simulink model "HANcoder_E407_DYS_MP"  (R2018b)
settings: Solver=FixedStepDiscrete  StartTime=0.0  StopTime=1  FixedStep=0.01  RelTol=1e-3
PreLoadFcn:
  | librarySetup
  | eval([bdroot,'_startup']) %Calling [modelName]_startup.m
values from neighbouring files (symbols this model uses):
  basic_cycle_duration_bc0 = TM_Reset_Board   + COMP_duration    (= 212)    [HANcoder_E407_DYS_MP_startup.m]
  basic_cycle_duration_bc1 = basic_cycle_duration_bc0    (= 212)    [HANcoder_E407_DYS_MP_startup.m]
  comm_delay_estimation1 = round(comm_delay_measured1*hardware_granularity/frequency_IRQ)    [HANcoder_E407_DYS_MP_startup.m]
  comm_delay_estimation2 = round(comm_delay_measured2*hardware_granularity/frequency_IRQ)    [HANcoder_E407_DYS_MP_startup.m]
  COMM_Phase1 = Simulink.Parameter    [HANcoder_E407_DYS_MP_startup.m]
  COMM_Phase2 = Simulink.Parameter    [HANcoder_E407_DYS_MP_startup.m]
  frequency_IRQ = 500    [HANcoder_E407_DYS_MP_startup.m]
  HantuneAngleSp = Simulink.Parameter    [HANcoder_E407_DYS_MP_startup.m]
  idle_time_init = basic_cycle_duration_bc0 + basic_cycle_duration_bc1    (= 424)    [HANcoder_E407_DYS_MP_startup.m]
  matrix_rows = 2    [HANcoder_E407_DYS_MP_startup.m]
  positionD = Simulink.Parameter    [HANcoder_E407_DYS_MP_startup.m]
  positionI = Simulink.Parameter    [HANcoder_E407_DYS_MP_startup.m]
  positionP = Simulink.Parameter    [HANcoder_E407_DYS_MP_startup.m]
undefined symbols (not defined in the file or in its folder): A1, CON2, CON4, D13, Dposition, Iposition, Pposition
libraries: HANcoder_STM32_Target x33, dspswit3 x16, simulink x2, simulink_extras x2, dspstat3 x1
(part 4 of 10)

== system HANcoder_E407_DYS_MP/HANcoder STM32 Target - E407-STM32 algorithm/4.TTA Can System/4.3 TTA System/4.3.3 Matrix Cycle Manager/4.3.3.1 Controller Matrix Cycle Truck Boards 1 2 and 3/4.3.3.1.1 controller basic cycle 0.1/Receive Timer can master message  ==
  Sender Id : Inport
  Enable : EnablePort  ShowOutputPort=on
  AND : Logic  Commented=on  IconShape=distinctive  AllPortsSameDT=off  OutDataTypeStr=boolean
  Constant : Constant  Value=100  OutDataTypeStr=uint32
  Constant1 : Constant  Value=10
  Constant2 : Constant  Value=2
  Constant3 : Constant  Commented=on  Value=6
  Constant4 : Constant  Commented=on  Value=16
  Constant5 : Constant  Commented=on  Value=26
  Constant6 : Constant  Commented=on  Value=36
  Constant7 : Constant  Commented=on  Value=46
  Counter : dspswit3/Counter  Direction=Up  CountEvent=Rising edge  CounterSize=User defined  MaxCount=255  InitialCount=0  Output=Count and Hit  HitValue=32  ResetInput=on  SamplesPerFrame=1  Ts=1  CntDtype=double  HitDtype=Logical
  Counter1 : dspswit3/Counter  Direction=Up  CountEvent=Rising edge  CounterSize=User defined  MaxCount=255  InitialCount=0  Output=Count and Hit  HitValue=32  ResetInput=on  SamplesPerFrame=1  Ts=1  CntDtype=double  HitDtype=Logical
  Counter2 : dspswit3/Counter  Direction=Up  CountEvent=Rising edge  CounterSize=User defined  MaxCount=255  InitialCount=0  Output=Count and Hit  HitValue=32  ResetInput=on  SamplesPerFrame=1  Ts=1  CntDtype=double  HitDtype=Logical
  Data Store Read1 : DataStoreRead  Commented=on  DataStoreName=Local_Ticks
  Data Store Read8 : DataStoreRead  DataStoreName=Local_Ticks
  Equal{,3..6} (5 alike) : RelationalOperator  Commented=on  Operator===  OutDataTypeStr=boolean  RndMeth=Simplest
  Equal1 : RelationalOperator  Operator===  OutDataTypeStr=boolean  RndMeth=Simplest
  Equal2 : RelationalOperator  Operator===  OutDataTypeStr=boolean  RndMeth=Simplest
  OR : Logic  Commented=on  Operator=OR  Inputs=5  IconShape=distinctive  AllPortsSameDT=off  OutDataTypeStr=boolean
  Receive can message : Subsystem  TreatAsAtomicUnit=on
  Terminator : Terminator
  Terminator1 : Terminator
  Terminator2 : Terminator
  Can1Mes : Outport
  Can1Rec : Outport  Port=2
  Can2Mes : Outport  Port=3
  Can2Rec : Outport  Port=4
  wires:
  Sender Id/1 -> Equal2/1
  Constant/1 -> Receive can message/1(Can_ID)
  Receive can message/1(Can1Port1) -> Can1Mes/1
  Receive can message/3(Can2Port2) -> Can2Mes/1
  Receive can message/2(Can1Receive) -> Counter1/1, Can1Rec/1
  Receive can message/4(Can2Receive) -> Can2Rec/1
  Equal1/1 -> Counter/1
  Counter/1 -> Terminator/1  "ReceiverTimerBlokCalls"
  Constant1/1 -> Equal1/2
  Data Store Read8/1 -> Equal1/1
  Counter1/1 -> Terminator1/1  "MessagesOnCan1"
  Constant2/1 -> Equal2/2
  Data Store Read1/1 -> Equal6/2, Equal5/2, Equal4/2, Equal3/2, Equal/2
  Constant6/1 -> Equal3/1
  OR/1 -> AND/1
  Constant7/1 -> Equal/1
  Equal2/1 -> Counter2/1, Receive can message/Enable
  Equal/1 -> OR/5
  Equal3/1 -> OR/4
  Constant5/1 -> Equal4/1
  Equal4/1 -> OR/3
  Constant4/1 -> Equal5/1
  Constant3/1 -> Equal6/1
  Equal6/1 -> OR/1
  Equal5/1 -> OR/2
  Counter2/1 -> Terminator2/1  "CanCallsCheck"

== system HANcoder_E407_DYS_MP/HANcoder STM32 Target - E407-STM32 algorithm/4.TTA Can System/4.3 TTA System/4.3.3 Matrix Cycle Manager/4.3.3.1 Controller Matrix Cycle Truck Boards 1 2 and 3/4.3.3.1.1 controller basic cycle 0.1/Receive Timer can master message 1 ==
  Input : Inport
  Enable : EnablePort  ShowOutputPort=on
  Desync calculation : Subsystem  Priority=10
  OR1 : Logic  Operator=OR  IconShape=distinctive  AllPortsSameDT=off  OutDataTypeStr=boolean
  Receive can message : Subsystem  TreatAsAtomicUnit=on
  Vote : Outport
  wires:
  Input/1 -> Receive can message/1(Can_ID)
  Enable/1 -> Receive can message/Enable
  OR1/1 -> Desync calculation/Enable
  Receive can message/4(Can2Receive) -> OR1/2
  Receive can message/2(Can1Receive) -> OR1/1, Desync calculation/1(New_msg_CAN1)
  Desync calculation/1(Vote) -> Vote/1
  Receive can message/3(Can2Port2) -> Desync calculation/3(Can2_Msg)
  Receive can message/1(Can1Port1) -> Desync calculation/2(Can1_Msg)

== system HANcoder_E407_DYS_MP/HANcoder STM32 Target - E407-STM32 algorithm/4.TTA Can System/4.3 TTA System/4.3.3 Matrix Cycle Manager/4.3.3.1 Controller Matrix Cycle Truck Boards 1 2 and 3/4.3.3.1.1 controller basic cycle 0.1/Receive Timer can master message 2 ==
  Input : Inport
  Enable : EnablePort  ShowOutputPort=on
  Desync calculation : Subsystem  Priority=10
  OR1 : Logic  Operator=OR  IconShape=distinctive  AllPortsSameDT=off  OutDataTypeStr=boolean
  Receive can message : Subsystem  TreatAsAtomicUnit=on
  Vote : Outport
  wires:
  Input/1 -> Receive can message/1(Can_ID)
  Enable/1 -> Receive can message/Enable
  OR1/1 -> Desync calculation/Enable
  Receive can message/4(Can2Receive) -> OR1/2
  Receive can message/2(Can1Receive) -> OR1/1, Desync calculation/1(New_msg_CAN1)
  Desync calculation/1(Vote) -> Vote/1
  Receive can message/3(Can2Port2) -> Desync calculation/3(Can2_Msg)
  Receive can message/1(Can1Port1) -> Desync calculation/2(Can1_Msg)

== system HANcoder_E407_DYS_MP/HANcoder STM32 Target - E407-STM32 algorithm/4.TTA Can System/4.3 TTA System/4.3.3 Matrix Cycle Manager/4.3.3.1 Controller Matrix Cycle Truck Boards 1 2 and 3/4.3.3.1.1 controller basic cycle 0.1/Receive Timer can master message 3 ==
  Input : Inport
  Enable : EnablePort  ShowOutputPort=on
  Desync calculation : Subsystem  Priority=10
  OR1 : Logic  Operator=OR  IconShape=distinctive  AllPortsSameDT=off  OutDataTypeStr=boolean
  Receive can message : Subsystem  TreatAsAtomicUnit=on
  Vote : Outport
  wires:
  Input/1 -> Receive can message/1(Can_ID)
  Enable/1 -> Receive can message/Enable
  OR1/1 -> Desync calculation/Enable
  Receive can message/4(Can2Receive) -> OR1/2
  Receive can message/2(Can1Receive) -> OR1/1, Desync calculation/1(New_msg_CAN1)
  Desync calculation/1(Vote) -> Vote/1
  Receive can message/3(Can2Port2) -> Desync calculation/3(Can2_Msg)
  Receive can message/1(Can1Port1) -> Desync calculation/2(Can1_Msg)

== system HANcoder_E407_DYS_MP/HANcoder STM32 Target - E407-STM32 algorithm/4.TTA Can System/4.3 TTA System/4.3.3 Matrix Cycle Manager/4.3.3.1 Controller Matrix Cycle Truck Boards 1 2 and 3/4.3.3.1.1 controller basic cycle 0.1/Send can message ==
  Can_ID : Inport
  Can_Data : Inport  Port=2
  Enable : EnablePort
  CAN send : Subsystem  Tag=HANcoder_TARGET_STM32_E407  AncestorBlock=HANcoder_STM32_Target/STM32-E407/CAN/CAN/CAN send  mask(CAN send){canBus=CAN 1, frameType=Standard (11 bit), inputNumber=1, dataType=uint8, byteOrder=on, tsamp=-1}
      mask prompts: canBus "CAN channel"; frameType "Identifier type"; inputNumber "Input ports"; dataType "Input datatype"; byteOrder "Byte order: Checked = MSB first, unchecked = LSB first."; tsamp "Sample time"
      mask help:
      | Function
      | ==========
      | Send a message on the CAN channel.
      |
      | Parameters
      | ==========
      | CAN channel:           The CAN channel to send the message on.
      | Identifier type:         normal or extended ID's
      | Input ports:              The amount of input ports
      | Input datatype:        The datatype of the input ports
      | Byte order:               Select MSB or LSB first
      | Sample time:            -1 or divisible by base sample time [seconds]
      |
      | Input
      | ==========
      | Port 1:                   CAN ID(uint32) in hexadecimal ie: hex2dec('0a')
      | Port 2..9                CAN message data
      mask init:
      | sfcn_can_send_mcb(canBus, frameType, inputNumber, dataType, byteOrder)
      settings: MoveFcn=drawLogos
      mask Help: web('sfcn_can_send.html');
      mask TypeOptions canBus: CAN 1 | CAN 2
      mask TypeOptions frameType: Standard (11 bit) | Extended (29 bit)
      mask TypeOptions dataType: int8 | uint8 | int16 | uint16 | int32 | uint32 | boolean
      mask Display:
      | fprintf('Send on\nCAN %x', canBus);
      | port_label('input', 1, 'ID');patch([105 111 111],[8 14 2],[1 0 0]);patch([113 113 119],[14 2 8],[0 0 0.35]);
  CAN send1 : Subsystem  Tag=HANcoder_TARGET_STM32_E407  AncestorBlock=HANcoder_STM32_Target/STM32-E407/CAN/CAN/CAN send  mask(CAN send){canBus=CAN 2, frameType=Standard (11 bit), inputNumber=1, dataType=uint8, byteOrder=on, tsamp=-1}
      mask prompts: canBus "CAN channel"; frameType "Identifier type"; inputNumber "Input ports"; dataType "Input datatype"; byteOrder "Byte order: Checked = MSB first, unchecked = LSB first."; tsamp "Sample time"
      mask help:
      | Function
      | ==========
      | Send a message on the CAN channel.
      |
      | Parameters
      | ==========
      | CAN channel:           The CAN channel to send the message on.
      | Identifier type:         normal or extended ID's
      | Input ports:              The amount of input ports
      | Input datatype:        The datatype of the input ports
      | Byte order:               Select MSB or LSB first
      | Sample time:            -1 or divisible by base sample time [seconds]
      |
      | Input
      | ==========
      | Port 1:                   CAN ID(uint32) in hexadecimal ie: hex2dec('0a')
      | Port 2..9                CAN message data
      mask init:
      | sfcn_can_send_mcb(canBus, frameType, inputNumber, dataType, byteOrder)
      settings: MoveFcn=drawLogos
      mask Help: web('sfcn_can_send.html');
      mask TypeOptions canBus: CAN 1 | CAN 2
      mask TypeOptions frameType: Standard (11 bit) | Extended (29 bit)
      mask TypeOptions dataType: int8 | uint8 | int16 | uint16 | int32 | uint32 | boolean
      mask Display:
      | fprintf('Send on\nCAN %x', canBus);
      | port_label('input', 1, 'ID');patch([105 111 111],[8 14 2],[1 0 0]);patch([113 113 119],[14 2 8],[0 0 0.35]);
  Cast To Double : DataTypeConversion  OutDataTypeStr=double
  Constant : Constant  Value=0
  Constant11 : Constant  Value=0
  Data Store Read10 : DataStoreRead  DataStoreName=VoteTime
  Data Store Write : DataStoreWrite  DataStoreName=Votes_count  DataStoreElements=Votes_count.First_Board
  Data Store Write1 : DataStoreWrite  DataStoreName=NoMes1
  Data Store Write2 : DataStoreWrite  Priority=23  DataStoreName=TwoTrailersAttachedFlag
  Data Store Write3 : DataStoreWrite  DataStoreName=TrailerOneAttachedFlag
  wires:
  Can_ID/1 -> CAN send1/1(In1), CAN send/1(In1)
  Can_Data/1 -> CAN send1/2(In2), CAN send/2(In2)
  Constant/1 -> Data Store Write3/1, Data Store Write2/1
  Constant11/1 -> Data Store Write1/1
  Data Store Read10/1 -> Cast To Double/1
  Cast To Double/1 -> Data Store Write/1

== system HANcoder_E407_DYS_MP/HANcoder STM32 Target - E407-STM32 algorithm/4.TTA Can System/4.3 TTA System/4.3.3 Matrix Cycle Manager/4.3.3.1 Controller Matrix Cycle Truck Boards 1 2 and 3/4.3.3.1.1 controller basic cycle 0.1/Send can message1 ==
  Can_ID : Inport
  Can_Data : Inport  Port=2
  Enable : EnablePort
  CAN send : Subsystem  Tag=HANcoder_TARGET_STM32_E407  AncestorBlock=HANcoder_STM32_Target/STM32-E407/CAN/CAN/CAN send  mask(CAN send){canBus=CAN 1, frameType=Standard (11 bit), inputNumber=1, dataType=uint8, byteOrder=on, tsamp=-1}
      mask prompts: canBus "CAN channel"; frameType "Identifier type"; inputNumber "Input ports"; dataType "Input datatype"; byteOrder "Byte order: Checked = MSB first, unchecked = LSB first."; tsamp "Sample time"
      mask help:
      | Function
      | ==========
      | Send a message on the CAN channel.
      |
      | Parameters
      | ==========
      | CAN channel:           The CAN channel to send the message on.
      | Identifier type:         normal or extended ID's
      | Input ports:              The amount of input ports
      | Input datatype:        The datatype of the input ports
      | Byte order:               Select MSB or LSB first
      | Sample time:            -1 or divisible by base sample time [seconds]
      |
      | Input
      | ==========
      | Port 1:                   CAN ID(uint32) in hexadecimal ie: hex2dec('0a')
      | Port 2..9                CAN message data
      mask init:
      | sfcn_can_send_mcb(canBus, frameType, inputNumber, dataType, byteOrder)
      settings: MoveFcn=drawLogos
      mask Help: web('sfcn_can_send.html');
      mask TypeOptions canBus: CAN 1 | CAN 2
      mask TypeOptions frameType: Standard (11 bit) | Extended (29 bit)
      mask TypeOptions dataType: int8 | uint8 | int16 | uint16 | int32 | uint32 | boolean
      mask Display:
      | fprintf('Send on\nCAN %x', canBus);
      | port_label('input', 1, 'ID');patch([105 111 111],[8 14 2],[1 0 0]);patch([113 113 119],[14 2 8],[0 0 0.35]);
  CAN send1 : Subsystem  Tag=HANcoder_TARGET_STM32_E407  AncestorBlock=HANcoder_STM32_Target/STM32-E407/CAN/CAN/CAN send  mask(CAN send){canBus=CAN 2, frameType=Standard (11 bit), inputNumber=1, dataType=uint8, byteOrder=on, tsamp=-1}
      mask prompts: canBus "CAN channel"; frameType "Identifier type"; inputNumber "Input ports"; dataType "Input datatype"; byteOrder "Byte order: Checked = MSB first, unchecked = LSB first."; tsamp "Sample time"
      mask help:
      | Function
      | ==========
      | Send a message on the CAN channel.
      |
      | Parameters
      | ==========
      | CAN channel:           The CAN channel to send the message on.
      | Identifier type:         normal or extended ID's
      | Input ports:              The amount of input ports
      | Input datatype:        The datatype of the input ports
      | Byte order:               Select MSB or LSB first
      | Sample time:            -1 or divisible by base sample time [seconds]
      |
      | Input
      | ==========
      | Port 1:                   CAN ID(uint32) in hexadecimal ie: hex2dec('0a')
      | Port 2..9                CAN message data
      mask init:
      | sfcn_can_send_mcb(canBus, frameType, inputNumber, dataType, byteOrder)
      settings: MoveFcn=drawLogos
      mask Help: web('sfcn_can_send.html');
      mask TypeOptions canBus: CAN 1 | CAN 2
      mask TypeOptions frameType: Standard (11 bit) | Extended (29 bit)
      mask TypeOptions dataType: int8 | uint8 | int16 | uint16 | int32 | uint32 | boolean
      mask Display:
      | fprintf('Send on\nCAN %x', canBus);
      | port_label('input', 1, 'ID');patch([105 111 111],[8 14 2],[1 0 0]);patch([113 113 119],[14 2 8],[0 0 0.35]);
  Cast To Double : DataTypeConversion  OutDataTypeStr=double
  Constant : Constant  Value=0
  Constant11 : Constant  Value=0
  Data Store Read10 : DataStoreRead  DataStoreName=VoteTime
  Data Store Write : DataStoreWrite  DataStoreName=Votes_count  DataStoreElements=Votes_count.Second_Board
  Data Store Write1 : DataStoreWrite  DataStoreName=NoMes2
  Data Store Write2 : DataStoreWrite  Priority=23  DataStoreName=TwoTrailersAttachedFlag
  Data Store Write3 : DataStoreWrite  DataStoreName=TrailerOneAttachedFlag
  wires:
  Can_ID/1 -> CAN send1/1(In1), CAN send/1(In1)
  Can_Data/1 -> CAN send1/2(In2), CAN send/2(In2)
  Constant11/1 -> Data Store Write1/1
  Data Store Read10/1 -> Cast To Double/1
  Cast To Double/1 -> Data Store Write/1
  Constant/1 -> Data Store Write3/1, Data Store Write2/1

== system HANcoder_E407_DYS_MP/HANcoder STM32 Target - E407-STM32 algorithm/4.TTA Can System/4.3 TTA System/4.3.3 Matrix Cycle Manager/4.3.3.1 Controller Matrix Cycle Truck Boards 1 2 and 3/4.3.3.1.1 controller basic cycle 0.1/Send can message2 ==
  Can_ID : Inport
  Can_Data : Inport  Port=2
  Enable : EnablePort
  CAN send : Subsystem  Tag=HANcoder_TARGET_STM32_E407  AncestorBlock=HANcoder_STM32_Target/STM32-E407/CAN/CAN/CAN send  mask(CAN send){canBus=CAN 1, frameType=Standard (11 bit), inputNumber=1, dataType=uint8, byteOrder=on, tsamp=-1}
      mask prompts: canBus "CAN channel"; frameType "Identifier type"; inputNumber "Input ports"; dataType "Input datatype"; byteOrder "Byte order: Checked = MSB first, unchecked = LSB first."; tsamp "Sample time"
      mask help:
      | Function
      | ==========
      | Send a message on the CAN channel.
      |
      | Parameters
      | ==========
      | CAN channel:           The CAN channel to send the message on.
      | Identifier type:         normal or extended ID's
      | Input ports:              The amount of input ports
      | Input datatype:        The datatype of the input ports
      | Byte order:               Select MSB or LSB first
      | Sample time:            -1 or divisible by base sample time [seconds]
      |
      | Input
      | ==========
      | Port 1:                   CAN ID(uint32) in hexadecimal ie: hex2dec('0a')
      | Port 2..9                CAN message data
      mask init:
      | sfcn_can_send_mcb(canBus, frameType, inputNumber, dataType, byteOrder)
      settings: MoveFcn=drawLogos
      mask Help: web('sfcn_can_send.html');
      mask TypeOptions canBus: CAN 1 | CAN 2
      mask TypeOptions frameType: Standard (11 bit) | Extended (29 bit)
      mask TypeOptions dataType: int8 | uint8 | int16 | uint16 | int32 | uint32 | boolean
      mask Display:
      | fprintf('Send on\nCAN %x', canBus);
      | port_label('input', 1, 'ID');patch([105 111 111],[8 14 2],[1 0 0]);patch([113 113 119],[14 2 8],[0 0 0.35]);
  CAN send1 : Subsystem  Tag=HANcoder_TARGET_STM32_E407  AncestorBlock=HANcoder_STM32_Target/STM32-E407/CAN/CAN/CAN send  mask(CAN send){canBus=CAN 2, frameType=Standard (11 bit), inputNumber=1, dataType=uint8, byteOrder=on, tsamp=-1}
      mask prompts: canBus "CAN channel"; frameType "Identifier type"; inputNumber "Input ports"; dataType "Input datatype"; byteOrder "Byte order: Checked = MSB first, unchecked = LSB first."; tsamp "Sample time"
      mask help:
      | Function
      | ==========
      | Send a message on the CAN channel.
      |
      | Parameters
      | ==========
      | CAN channel:           The CAN channel to send the message on.
      | Identifier type:         normal or extended ID's
      | Input ports:              The amount of input ports
      | Input datatype:        The datatype of the input ports
      | Byte order:               Select MSB or LSB first
      | Sample time:            -1 or divisible by base sample time [seconds]
      |
      | Input
      | ==========
      | Port 1:                   CAN ID(uint32) in hexadecimal ie: hex2dec('0a')
      | Port 2..9                CAN message data
      mask init:
      | sfcn_can_send_mcb(canBus, frameType, inputNumber, dataType, byteOrder)
      settings: MoveFcn=drawLogos
      mask Help: web('sfcn_can_send.html');
      mask TypeOptions canBus: CAN 1 | CAN 2
      mask TypeOptions frameType: Standard (11 bit) | Extended (29 bit)
      mask TypeOptions dataType: int8 | uint8 | int16 | uint16 | int32 | uint32 | boolean
      mask Display:
      | fprintf('Send on\nCAN %x', canBus);
      | port_label('input', 1, 'ID');patch([105 111 111],[8 14 2],[1 0 0]);patch([113 113 119],[14 2 8],[0 0 0.35]);
  Cast To Double : DataTypeConversion  OutDataTypeStr=double
  Constant : Constant  Value=0
  Constant11 : Constant  Value=0
  Data Store Read10 : DataStoreRead  DataStoreName=VoteTime
  Data Store Write : DataStoreWrite  DataStoreName=Votes_count  DataStoreElements=Votes_count.Third_Board
  Data Store Write1 : DataStoreWrite  DataStoreName=NoMes3
  Data Store Write2 : DataStoreWrite  Priority=23  DataStoreName=TwoTrailersAttachedFlag
  Data Store Write3 : DataStoreWrite  DataStoreName=TrailerOneAttachedFlag
  wires:
  Can_ID/1 -> CAN send1/1(In1), CAN send/1(In1)
  Can_Data/1 -> CAN send1/2(In2), CAN send/2(In2)
  Constant11/1 -> Data Store Write1/1
  Data Store Read10/1 -> Cast To Double/1
  Cast To Double/1 -> Data Store Write/1
  Constant/1 -> Data Store Write3/1, Data Store Write2/1

== system HANcoder_E407_DYS_MP/HANcoder STM32 Target - E407-STM32 algorithm/4.TTA Can System/4.3 TTA System/4.3.3 Matrix Cycle Manager/4.3.3.1 Controller Matrix Cycle Truck Boards 1 2 and 3/4.3.3.1.1 controller basic cycle 0.1/Send//Receive Timer can master message  ==
  Sender Id : Inport
  Can_Data : Inport  Port=2
  Enable : EnablePort  ShowOutputPort=on
  Constant : Constant  Value=100  OutDataTypeStr=uint32
  If : If  IfExpression=u1 == 1  ElseIfExpressions=(u1 > 1) & (u1 <= 3)
  Send can message : Subsystem  TreatAsAtomicUnit=on
  wires:
  Can_Data/1 -> Send can message/2(Can_Data)  "CanSendTime"
  Sender Id/1 -> If/1
  If/1 -> Send can message/Action
  Constant/1 -> Send can message/1(Can_ID)

== system HANcoder_E407_DYS_MP/HANcoder STM32 Target - E407-STM32 algorithm/4.TTA Can System/4.3 TTA System/4.3.3 Matrix Cycle Manager/4.3.3.1 Controller Matrix Cycle Truck Boards 1 2 and 3/4.3.3.1.2 controller basic cycle 0.2/If Action Subsystem ==
  Enable : EnablePort  ShowOutputPort=on
  Constant : Constant
  Constant1 : Constant  Value=0
  Constant2 : Constant  Value=90
  Constant3 : Constant  Value=0
  Constant35 : Constant  Priority=22  Value=HantuneAngleSp
  Constant4 : Constant
  Data Store Read1 : DataStoreRead  DataStoreName=InputAngle1
  Data Store Read15 : DataStoreRead  DataStoreName=TwoTrailersAttachedFlag
  Data Store Read2 : DataStoreRead  DataStoreName=InputAngle2
  Data Store Read3 : DataStoreRead  DataStoreName=TrailerOneAttachedFlag
  Data Store Write1 : DataStoreWrite  Priority=23  DataStoreName=CalcSteeringAngle
  Data Store Write2 : DataStoreWrite  Priority=23  DataStoreName=NoTrailerAttachError
  Degrees to Radians : simulink_extras/Transformations/Degrees to Radians
  Equal : RelationalOperator  Operator===  OutDataTypeStr=boolean  RndMeth=Simplest
  Equal1 : RelationalOperator  Operator===  OutDataTypeStr=boolean  RndMeth=Simplest
  Radians to Degrees : simulink_extras/Transformations/Radians to Degrees
  Subsystem : Subsystem
  Subtract : Sum  Inputs=+-
  Subtract1 : Sum  Inputs=+-
  Subtract2 : Sum  Inputs=+-
  Switch : Switch  Criteria=u2 > Threshold
  Switch1 : Switch  Criteria=u2 > Threshold
  Switch2 : Switch  Criteria=u2 > Threshold
  wires:
  Data Store Read15/1 -> Equal/1
  Constant/1 -> Equal/2
  Equal/1 -> Switch/2, Switch1/2
  Constant1/1 -> Switch/3
  Subtract1/1 -> Switch1/3, Switch/1
  Subsystem/1(delta_12K) -> Radians to Degrees/1
  Degrees to Radians/1 -> Subsystem/3(delta_c)
  Switch1/1 -> Degrees to Radians/1
  Radians to Degrees/1 -> Data Store Write1/1
  Switch/1 -> Subsystem/1(Gamma2)
  Constant35/1 -> Subtract2/1
  Data Store Read1/1 -> Subtract1/1
  Constant2/1 -> Subtract1/2, Subtract2/2, Subtract/2
  Data Store Read2/1 -> Subtract/1
  Subtract/1 -> Switch1/1
  Subtract2/1 -> Subsystem/2(Gamma1)
  Constant3/1 -> Switch2/3, Equal1/2
  Data Store Read3/1 -> Equal1/1
  Equal1/1 -> Switch2/2
  Switch2/1 -> Data Store Write2/1
  Constant4/1 -> Switch2/1

== system HANcoder_E407_DYS_MP/HANcoder STM32 Target - E407-STM32 algorithm/4.TTA Can System/4.3 TTA System/4.3.3 Matrix Cycle Manager/4.3.3.1 Controller Matrix Cycle Truck Boards 1 2 and 3/4.3.3.1.2 controller basic cycle 0.2/If Action Subsystem1 ==
  Enable : EnablePort  ShowOutputPort=on
  AND : Logic  IconShape=distinctive  AllPortsSameDT=off  OutDataTypeStr=boolean
  AND1 : Logic  IconShape=distinctive  AllPortsSameDT=off  OutDataTypeStr=boolean
  AND2 : Logic  IconShape=distinctive  AllPortsSameDT=off  OutDataTypeStr=boolean
  AND3 : Logic  Operator=NOR  Inputs=3  IconShape=distinctive  AllPortsSameDT=off  OutDataTypeStr=boolean
  Add : Sum
  Add1 : Sum  Inputs=-+
  Add4 : Sum
  Add5 : Sum  Inputs=-+
  Constant : Constant  Value=0.005
  Constant1 : Constant
  Constant2 : Constant  Value=0
  Constant3 : Constant  Value=0
  Data Store Read17 : DataStoreRead  DataStoreName=Votes_Angle  DataStoreElements=Votes_Angle.First_Board#Votes_Angle.Second_Board#Votes_Angle.Third_Board
  Data Store Write1 : DataStoreWrite  Priority=23  DataStoreName=ValitdatedSteeringAngle
  Data Store Write2 : DataStoreWrite  Priority=23  DataStoreName=AngleVoteError
  GreaterThanOrEqual : RelationalOperator  Operator=<  OutDataTypeStr=boolean  RndMeth=Simplest
  GreaterThanOrEqual1 : RelationalOperator  Operator=>  OutDataTypeStr=boolean  RndMeth=Simplest
  GreaterThanOrEqual2 : RelationalOperator  OutDataTypeStr=boolean  RndMeth=Simplest
  GreaterThanOrEqual3 : RelationalOperator  Operator=<=  OutDataTypeStr=boolean  RndMeth=Simplest
  GreaterThanOrEqual4 : RelationalOperator  OutDataTypeStr=boolean  RndMeth=Simplest
  GreaterThanOrEqual5 : RelationalOperator  Operator=<=  OutDataTypeStr=boolean  RndMeth=Simplest
  Switch{,1..3} (4 alike) : Switch  Criteria=u2 > Threshold
  wires:
  Data Store Read17/2 -> GreaterThanOrEqual1/2, GreaterThanOrEqual/2, GreaterThanOrEqual2/1, GreaterThanOrEqual3/1, Switch2/1
  Constant/1 -> Add/2, Add5/1, Add4/2, Add1/1
  Data Store Read17/3 -> Add5/2, Add4/1
  Add1/1 -> GreaterThanOrEqual/1
  Add/1 -> GreaterThanOrEqual1/1
  GreaterThanOrEqual3/1 -> AND/1
  GreaterThanOrEqual2/1 -> AND/2
  GreaterThanOrEqual1/1 -> AND1/1
  GreaterThanOrEqual/1 -> AND1/2
  AND1/1 -> AND3/1, Switch/2
  Switch1/1 -> Switch/3
  Data Store Read17/1 -> GreaterThanOrEqual4/1, GreaterThanOrEqual5/1, Switch1/1, Switch/1, Add1/2, Add/1
  Add4/1 -> GreaterThanOrEqual5/2, GreaterThanOrEqual3/2
  GreaterThanOrEqual4/1 -> AND2/2
  GreaterThanOrEqual5/1 -> AND2/1
  Add5/1 -> GreaterThanOrEqual4/2, GreaterThanOrEqual2/2
  Switch2/1 -> Switch1/3
  AND/1 -> AND3/3, Switch2/2
  Constant3/1 -> Switch2/3
  Switch/1 -> Data Store Write1/1
  AND2/1 -> Switch1/2, AND3/2
  AND3/1 -> Switch3/2
  Constant1/1 -> Switch3/1
  Switch3/1 -> Data Store Write2/1
  Constant2/1 -> Switch3/3

== system HANcoder_E407_DYS_MP/HANcoder STM32 Target - E407-STM32 algorithm/4.TTA Can System/4.3 TTA System/4.3.3 Matrix Cycle Manager/4.3.3.1 Controller Matrix Cycle Truck Boards 1 2 and 3/4.3.3.1.2 controller basic cycle 0.2/If Action Subsystem2 ==
  Enable : EnablePort  ShowOutputPort=on
  AND : Logic  IconShape=distinctive  AllPortsSameDT=off  OutDataTypeStr=boolean
  Constant : Constant
  Data Store Read : DataStoreRead  DataStoreName=AngleVoteError
  Data Store Read1 : DataStoreRead  DataStoreName=Role_ID
  Equal : RelationalOperator  Operator===  OutDataTypeStr=boolean  RndMeth=Simplest
  If Action Subsystem2 : Subsystem  TreatAsAtomicUnit=on
  NOT : Logic  Operator=NOT  IconShape=distinctive  AllPortsSameDT=off  OutDataTypeStr=boolean
  wires:
  Data Store Read/1 -> NOT/1
  NOT/1 -> AND/2
  Data Store Read1/1 -> Equal/1
  Constant/1 -> Equal/2
  Equal/1 -> AND/1
  AND/1 -> If Action Subsystem2/Enable

== system HANcoder_E407_DYS_MP/HANcoder STM32 Target - E407-STM32 algorithm/4.TTA Can System/4.3 TTA System/4.3.3 Matrix Cycle Manager/4.3.3.1 Controller Matrix Cycle Truck Boards 1 2 and 3/4.3.3.1.2 controller basic cycle 0.2/If Action Subsystem3 ==
  note: CAN ID Init
  Enable : EnablePort  ShowOutputPort=on
  Add : Sum  Inputs=+++
  Constant : Constant
  Constant1 : Constant  Value=2
  Constant2 : Constant  Value=4
  Constant3 : Constant
  Constant4 : Constant  Value=0
  Data Store Read20 : DataStoreRead  DataStoreName=Board_ID
  Data Store Write : DataStoreWrite  DataStoreName=BoardIdError
  Digital Input4 : HANcoder_STM32_Target/STM32-E407/Digital Inputs/Digital Input  Tag=HANcoder_TARGET_STM32_E407  pinID=CON3 - D2 - 5V Tolerant  config=Pulldown  tsamp=-1
      settings: SourceProductName=HANcoder STM32 Target
  Digital Input5 : HANcoder_STM32_Target/STM32-E407/Digital Inputs/Digital Input  Tag=HANcoder_TARGET_STM32_E407  pinID=CON3 - D3 - 5V Tolerant  config=Pulldown  tsamp=-1
      settings: SourceProductName=HANcoder STM32 Target
  Digital Input6 : HANcoder_STM32_Target/STM32-E407/Digital Inputs/Digital Input  Tag=HANcoder_TARGET_STM32_E407  pinID=CON3 - D4 - 5V Tolerant  config=Pulldown  tsamp=-1
      settings: SourceProductName=HANcoder STM32 Target
  Equal : RelationalOperator  Operator===  OutDataTypeStr=boolean  RndMeth=Simplest
  Multiply : Product
  Multiply1 : Product
  Multiply2 : Product
  Switch : Switch  Criteria=u2 > Threshold
  wires:
  Multiply1/1 -> Add/2
  Multiply2/1 -> Add/3
  Constant/1 -> Multiply/1
  Constant1/1 -> Multiply1/1
  Digital Input6/1 -> Multiply2/2
  Digital Input5/1 -> Multiply1/2
  Multiply/1 -> Add/1
  Constant2/1 -> Multiply2/1
  Digital Input4/1 -> Multiply/2
  Add/1 -> Equal/2
  Data Store Read20/1 -> Equal/1
  Equal/1 -> Switch/2
  Constant3/1 -> Switch/3
  Constant4/1 -> Switch/1
  Switch/1 -> Data Store Write/1

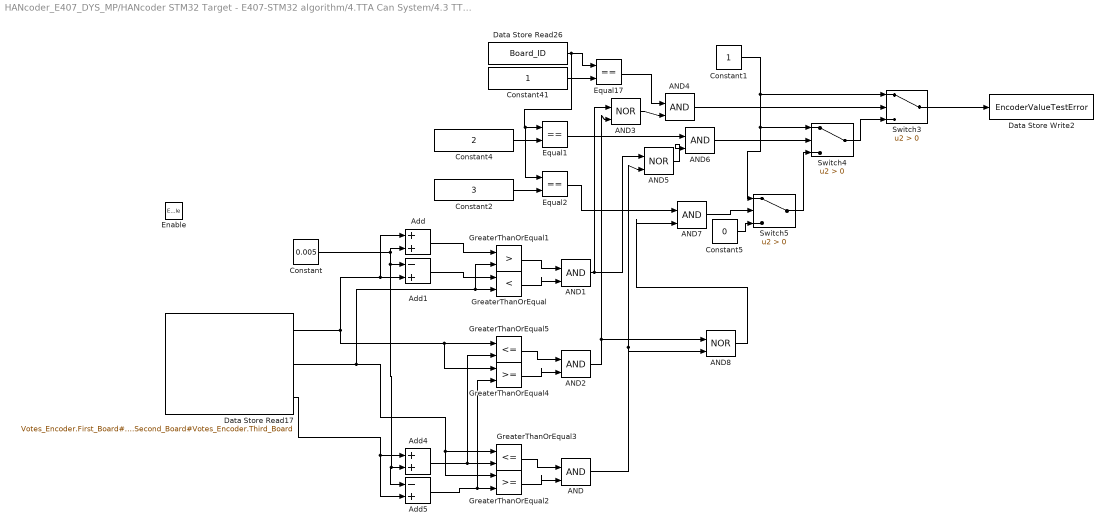
== system HANcoder_E407_DYS_MP/HANcoder STM32 Target - E407-STM32 algorithm/4.TTA Can System/4.3 TTA System/4.3.3 Matrix Cycle Manager/4.3.3.1 Controller Matrix Cycle Truck Boards 1 2 and 3/4.3.3.1.2 controller basic cycle 0.2/If Action Subsystem4 ==
  Enable : EnablePort  ShowOutputPort=on
  AND{,1..2,4,6..7} (6 alike) : Logic  IconShape=distinctive  AllPortsSameDT=off  OutDataTypeStr=boolean
  AND3 : Logic  Operator=NOR  IconShape=distinctive  AllPortsSameDT=off  OutDataTypeStr=boolean
  AND5 : Logic  Operator=NOR  IconShape=distinctive  AllPortsSameDT=off  OutDataTypeStr=boolean
  AND8 : Logic  Operator=NOR  IconShape=distinctive  AllPortsSameDT=off  OutDataTypeStr=boolean
  Add : Sum
  Add1 : Sum  Inputs=-+
  Add4 : Sum
  Add5 : Sum  Inputs=-+
  Constant : Constant  Value=0.005
  Constant1 : Constant
  Constant2 : Constant  Value=3
  Constant4 : Constant  Value=2
  Constant41 : Constant
  Constant5 : Constant  Value=0
  Data Store Read17 : DataStoreRead  DataStoreName=Votes_Encoder  DataStoreElements=Votes_Encoder.First_Board#Votes_Encoder.Second_Board#Votes_Encoder.Third_Board
  Data Store Read26 : DataStoreRead  DataStoreName=Board_ID
  Data Store Write2 : DataStoreWrite  Priority=23  DataStoreName=EncoderValueTestError
  Equal1 : RelationalOperator  Operator===  OutDataTypeStr=boolean  RndMeth=Simplest
  Equal17 : RelationalOperator  Operator===  OutDataTypeStr=boolean  RndMeth=Simplest
  Equal2 : RelationalOperator  Operator===  OutDataTypeStr=boolean  RndMeth=Simplest
  GreaterThanOrEqual : RelationalOperator  Operator=<  OutDataTypeStr=boolean  RndMeth=Simplest
  GreaterThanOrEqual1 : RelationalOperator  Operator=>  OutDataTypeStr=boolean  RndMeth=Simplest
  GreaterThanOrEqual2 : RelationalOperator  OutDataTypeStr=boolean  RndMeth=Simplest
  GreaterThanOrEqual3 : RelationalOperator  Operator=<=  OutDataTypeStr=boolean  RndMeth=Simplest
  GreaterThanOrEqual4 : RelationalOperator  OutDataTypeStr=boolean  RndMeth=Simplest
  GreaterThanOrEqual5 : RelationalOperator  Operator=<=  OutDataTypeStr=boolean  RndMeth=Simplest
  Switch3 : Switch  Criteria=u2 > Threshold
  Switch4 : Switch  Criteria=u2 > Threshold
  Switch5 : Switch  Criteria=u2 > Threshold
  wires:
  Data Store Read17/2 -> GreaterThanOrEqual1/2, GreaterThanOrEqual/2, GreaterThanOrEqual2/1, GreaterThanOrEqual3/1
  Constant/1 -> Add/2, Add5/1, Add4/2, Add1/1
  Data Store Read17/3 -> Add5/2, Add4/1
  Add1/1 -> GreaterThanOrEqual/1
  Add/1 -> GreaterThanOrEqual1/1
  GreaterThanOrEqual3/1 -> AND/1
  GreaterThanOrEqual2/1 -> AND/2
  GreaterThanOrEqual1/1 -> AND1/1
  GreaterThanOrEqual/1 -> AND1/2
  AND1/1 -> AND3/1, AND5/1
  Data Store Read17/1 -> GreaterThanOrEqual4/1, GreaterThanOrEqual5/1, Add1/2, Add/1
  Add4/1 -> GreaterThanOrEqual5/2, GreaterThanOrEqual3/2
  GreaterThanOrEqual4/1 -> AND2/2
  GreaterThanOrEqual5/1 -> AND2/1
  Add5/1 -> GreaterThanOrEqual4/2, GreaterThanOrEqual2/2
  AND/1 -> AND8/2, AND5/2
  AND2/1 -> AND8/1, AND3/2
  Constant1/1 -> Switch5/1, Switch4/1, Switch3/1
  Switch3/1 -> Data Store Write2/1
  Switch4/1 -> Switch3/3
  Constant41/1 -> Equal17/2
  AND3/1 -> AND4/2
  Equal17/1 -> AND4/1
  AND4/1 -> Switch3/2
  Data Store Read26/1 -> Equal2/1, Equal1/1, Equal17/1
  Constant4/1 -> Equal1/2
  AND5/1 -> AND6/2
  Equal1/1 -> AND6/1
  AND6/1 -> Switch4/2
  Constant2/1 -> Equal2/2
  Switch5/1 -> Switch4/3
  Constant5/1 -> Switch5/3
  AND7/1 -> Switch5/2
  Equal2/1 -> AND7/1
  AND8/1 -> AND7/2

== system HANcoder_E407_DYS_MP/HANcoder STM32 Target - E407-STM32 algorithm/4.TTA Can System/4.3 TTA System/4.3.3 Matrix Cycle Manager/4.3.3.1 Controller Matrix Cycle Truck Boards 1 2 and 3/4.3.3.1.2 controller basic cycle 0.2/Receive Trailer 1 board 4 input angel ==
  Input : Inport
  Enable : EnablePort  ShowOutputPort=on
  Desync calculation : Subsystem  Priority=10
  OR1 : Logic  Operator=OR  IconShape=distinctive  AllPortsSameDT=off  OutDataTypeStr=boolean
  Receive can message : Subsystem  TreatAsAtomicUnit=on
  Angle : Outport
  wires:
  Input/1 -> Receive can message/1(Can_ID)
  Enable/1 -> Receive can message/Enable
  OR1/1 -> Desync calculation/Enable
  Receive can message/4(Can2Receive) -> OR1/2
  Receive can message/2(Can1Receive) -> OR1/1, Desync calculation/1(New_msg_CAN1)
  Desync calculation/1(Vote) -> Angle/1
  Receive can message/3(Can2Port2) -> Desync calculation/3(Can2_Msg)
  Receive can message/1(Can1Port1) -> Desync calculation/2(Can1_Msg)

== system HANcoder_E407_DYS_MP/HANcoder STM32 Target - E407-STM32 algorithm/4.TTA Can System/4.3 TTA System/4.3.3 Matrix Cycle Manager/4.3.3.1 Controller Matrix Cycle Truck Boards 1 2 and 3/4.3.3.1.2 controller basic cycle 0.2/Receive Trailer 2 board 5 input angel ==
  Input : Inport
  Enable : EnablePort  ShowOutputPort=on
  OR1 : Logic  Operator=OR  IconShape=distinctive  AllPortsSameDT=off  OutDataTypeStr=boolean
  Receive Mes : Subsystem  Priority=10
  Receive can message : Subsystem  TreatAsAtomicUnit=on
  Angle : Outport
  wires:
  Input/1 -> Receive can message/1(Can_ID)
  Enable/1 -> Receive can message/Enable
  OR1/1 -> Receive Mes/Enable
  Receive can message/4(Can2Receive) -> OR1/2
  Receive can message/2(Can1Receive) -> OR1/1, Receive Mes/1(New_msg_CAN1)
  Receive Mes/1(Vote) -> Angle/1
  Receive can message/3(Can2Port2) -> Receive Mes/3(Can2_Msg)
  Receive can message/1(Can1Port1) -> Receive Mes/2(Can1_Msg)

== system HANcoder_E407_DYS_MP/HANcoder STM32 Target - E407-STM32 algorithm/4.TTA Can System/4.3 TTA System/4.3.3 Matrix Cycle Manager/4.3.3.1 Controller Matrix Cycle Truck Boards 1 2 and 3/4.3.3.1.2 controller basic cycle 0.2/Receive Truck 1 Board 1 Calc Steering Angle ==
  Input : Inport
  Enable : EnablePort  ShowOutputPort=on
  Desync calculation : Subsystem  Priority=10
  OR1 : Logic  Operator=OR  IconShape=distinctive  AllPortsSameDT=off  OutDataTypeStr=boolean
  Receive can message : Subsystem  TreatAsAtomicUnit=on
  Angle : Outport
  wires:
  Input/1 -> Receive can message/1(Can_ID)
  Enable/1 -> Receive can message/Enable
  OR1/1 -> Desync calculation/Enable
  Receive can message/4(Can2Receive) -> OR1/2
  Receive can message/2(Can1Receive) -> OR1/1, Desync calculation/1(New_msg_CAN1)
  Desync calculation/1(Vote) -> Angle/1
  Receive can message/3(Can2Port2) -> Desync calculation/3(Can2_Msg)
  Receive can message/1(Can1Port1) -> Desync calculation/2(Can1_Msg)

== system HANcoder_E407_DYS_MP/HANcoder STM32 Target - E407-STM32 algorithm/4.TTA Can System/4.3 TTA System/4.3.3 Matrix Cycle Manager/4.3.3.1 Controller Matrix Cycle Truck Boards 1 2 and 3/4.3.3.1.2 controller basic cycle 0.2/Receive Truck 1 Board 1 Calc Steering Angle1 ==
  Input : Inport
  Enable : EnablePort  ShowOutputPort=on
  Desync calculation : Subsystem  Priority=10
  OR1 : Logic  Operator=OR  IconShape=distinctive  AllPortsSameDT=off  OutDataTypeStr=boolean
  Receive can message : Subsystem  TreatAsAtomicUnit=on
  Angle : Outport
  wires:
  Input/1 -> Receive can message/1(Can_ID)
  Enable/1 -> Receive can message/Enable
  OR1/1 -> Desync calculation/Enable
  Receive can message/4(Can2Receive) -> OR1/2
  Receive can message/2(Can1Receive) -> OR1/1, Desync calculation/1(New_msg_CAN1)
  Desync calculation/1(Vote) -> Angle/1
  Receive can message/3(Can2Port2) -> Desync calculation/3(Can2_Msg)
  Receive can message/1(Can1Port1) -> Desync calculation/2(Can1_Msg)

== system HANcoder_E407_DYS_MP/HANcoder STM32 Target - E407-STM32 algorithm/4.TTA Can System/4.3 TTA System/4.3.3 Matrix Cycle Manager/4.3.3.1 Controller Matrix Cycle Truck Boards 1 2 and 3/4.3.3.1.2 controller basic cycle 0.2/Receive Truck 1 Board 1 Calc Steering Angle2 ==
  Input : Inport
  Enable : EnablePort  ShowOutputPort=on
  Desync calculation : Subsystem  Priority=10
  OR1 : Logic  Operator=OR  IconShape=distinctive  AllPortsSameDT=off  OutDataTypeStr=boolean
  Receive can message : Subsystem  TreatAsAtomicUnit=on
  Angle : Outport
  wires:
  Input/1 -> Receive can message/1(Can_ID)
  Enable/1 -> Receive can message/Enable
  OR1/1 -> Desync calculation/Enable
  Receive can message/4(Can2Receive) -> OR1/2
  Receive can message/2(Can1Receive) -> OR1/1, Desync calculation/1(New_msg_CAN1)
  Desync calculation/1(Vote) -> Angle/1
  Receive can message/3(Can2Port2) -> Desync calculation/3(Can2_Msg)
  Receive can message/1(Can1Port1) -> Desync calculation/2(Can1_Msg)

== system HANcoder_E407_DYS_MP/HANcoder STM32 Target - E407-STM32 algorithm/4.TTA Can System/4.3 TTA System/4.3.3 Matrix Cycle Manager/4.3.3.1 Controller Matrix Cycle Truck Boards 1 2 and 3/4.3.3.1.2 controller basic cycle 0.2/Receive Truck 1 Board 1 Calc Steering Angle3 ==
  Input : Inport
  Enable : EnablePort  ShowOutputPort=on
  Desync calculation : Subsystem  Priority=10
  OR1 : Logic  Operator=OR  IconShape=distinctive  AllPortsSameDT=off  OutDataTypeStr=boolean
  Receive can message : Subsystem  TreatAsAtomicUnit=on
  Angle : Outport
  wires:
  Input/1 -> Receive can message/1(Can_ID)
  Enable/1 -> Receive can message/Enable
  OR1/1 -> Desync calculation/Enable
  Receive can message/4(Can2Receive) -> OR1/2
  Receive can message/2(Can1Receive) -> OR1/1, Desync calculation/1(New_msg_CAN1)
  Desync calculation/1(Vote) -> Angle/1
  Receive can message/3(Can2Port2) -> Desync calculation/3(Can2_Msg)
  Receive can message/1(Can1Port1) -> Desync calculation/2(Can1_Msg)

== system HANcoder_E407_DYS_MP/HANcoder STM32 Target - E407-STM32 algorithm/4.TTA Can System/4.3 TTA System/4.3.3 Matrix Cycle Manager/4.3.3.1 Controller Matrix Cycle Truck Boards 1 2 and 3/4.3.3.1.2 controller basic cycle 0.2/Receive Truck 2 Board 2 Calc Steering Angle ==
  Input : Inport
  Enable : EnablePort  ShowOutputPort=on
  Desync calculation : Subsystem  Priority=10
  OR1 : Logic  Operator=OR  IconShape=distinctive  AllPortsSameDT=off  OutDataTypeStr=boolean
  Receive can message : Subsystem  TreatAsAtomicUnit=on
  Angle : Outport
  wires:
  Input/1 -> Receive can message/1(Can_ID)
  Enable/1 -> Receive can message/Enable
  OR1/1 -> Desync calculation/Enable
  Receive can message/4(Can2Receive) -> OR1/2
  Receive can message/2(Can1Receive) -> OR1/1, Desync calculation/1(New_msg_CAN1)
  Desync calculation/1(Vote) -> Angle/1
  Receive can message/3(Can2Port2) -> Desync calculation/3(Can2_Msg)
  Receive can message/1(Can1Port1) -> Desync calculation/2(Can1_Msg)

== system HANcoder_E407_DYS_MP/HANcoder STM32 Target - E407-STM32 algorithm/4.TTA Can System/4.3 TTA System/4.3.3 Matrix Cycle Manager/4.3.3.1 Controller Matrix Cycle Truck Boards 1 2 and 3/4.3.3.1.2 controller basic cycle 0.2/Receive Truck 3 Board 3 Calc Steering Angle ==
  Input : Inport
  Enable : EnablePort  ShowOutputPort=on
  Desync calculation : Subsystem  Priority=10
  OR1 : Logic  Operator=OR  IconShape=distinctive  AllPortsSameDT=off  OutDataTypeStr=boolean
  Receive can message : Subsystem  TreatAsAtomicUnit=on
  Angle : Outport
  wires:
  Input/1 -> Receive can message/1(Can_ID)
  Enable/1 -> Receive can message/Enable
  OR1/1 -> Desync calculation/Enable
  Receive can message/4(Can2Receive) -> OR1/2
  Receive can message/2(Can1Receive) -> OR1/1, Desync calculation/1(New_msg_CAN1)
  Desync calculation/1(Vote) -> Angle/1
  Receive can message/3(Can2Port2) -> Desync calculation/3(Can2_Msg)
  Receive can message/1(Can1Port1) -> Desync calculation/2(Can1_Msg)

== system HANcoder_E407_DYS_MP/HANcoder STM32 Target - E407-STM32 algorithm/4.TTA Can System/4.3 TTA System/4.3.3 Matrix Cycle Manager/4.3.3.1 Controller Matrix Cycle Truck Boards 1 2 and 3/4.3.3.1.2 controller basic cycle 0.2/Send can message ==
  Can_ID : Inport
  Can_Data : Inport  Port=2
  Enable : EnablePort
  CAN send : Subsystem  Tag=HANcoder_TARGET_STM32_E407  AncestorBlock=HANcoder_STM32_Target/STM32-E407/CAN/CAN/CAN send  mask(CAN send){canBus=CAN 1, frameType=Standard (11 bit), inputNumber=1, dataType=uint8, byteOrder=on, tsamp=-1}
      mask prompts: canBus "CAN channel"; frameType "Identifier type"; inputNumber "Input ports"; dataType "Input datatype"; byteOrder "Byte order: Checked = MSB first, unchecked = LSB first."; tsamp "Sample time"
      mask help:
      | Function
      | ==========
      | Send a message on the CAN channel.
      |
      | Parameters
      | ==========
      | CAN channel:           The CAN channel to send the message on.
      | Identifier type:         normal or extended ID's
      | Input ports:              The amount of input ports
      | Input datatype:        The datatype of the input ports
      | Byte order:               Select MSB or LSB first
      | Sample time:            -1 or divisible by base sample time [seconds]
      |
      | Input
      | ==========
      | Port 1:                   CAN ID(uint32) in hexadecimal ie: hex2dec('0a')
      | Port 2..9                CAN message data
      mask init:
      | sfcn_can_send_mcb(canBus, frameType, inputNumber, dataType, byteOrder)
      settings: MoveFcn=drawLogos
      mask Help: web('sfcn_can_send.html');
      mask TypeOptions canBus: CAN 1 | CAN 2
      mask TypeOptions frameType: Standard (11 bit) | Extended (29 bit)
      mask TypeOptions dataType: int8 | uint8 | int16 | uint16 | int32 | uint32 | boolean
      mask Display:
      | fprintf('Send on\nCAN %x', canBus);
      | port_label('input', 1, 'ID');patch([105 111 111],[8 14 2],[1 0 0]);patch([113 113 119],[14 2 8],[0 0 0.35]);
  CAN send1 : Subsystem  Tag=HANcoder_TARGET_STM32_E407  AncestorBlock=HANcoder_STM32_Target/STM32-E407/CAN/CAN/CAN send  mask(CAN send){canBus=CAN 2, frameType=Standard (11 bit), inputNumber=1, dataType=uint8, byteOrder=on, tsamp=-1}
      mask prompts: canBus "CAN channel"; frameType "Identifier type"; inputNumber "Input ports"; dataType "Input datatype"; byteOrder "Byte order: Checked = MSB first, unchecked = LSB first."; tsamp "Sample time"
      mask help:
      | Function
      | ==========
      | Send a message on the CAN channel.
      |
      | Parameters
      | ==========
      | CAN channel:           The CAN channel to send the message on.
      | Identifier type:         normal or extended ID's
      | Input ports:              The amount of input ports
      | Input datatype:        The datatype of the input ports
      | Byte order:               Select MSB or LSB first
      | Sample time:            -1 or divisible by base sample time [seconds]
      |
      | Input
      | ==========
      | Port 1:                   CAN ID(uint32) in hexadecimal ie: hex2dec('0a')
      | Port 2..9                CAN message data
      mask init:
      | sfcn_can_send_mcb(canBus, frameType, inputNumber, dataType, byteOrder)
      settings: MoveFcn=drawLogos
      mask Help: web('sfcn_can_send.html');
      mask TypeOptions canBus: CAN 1 | CAN 2
      mask TypeOptions frameType: Standard (11 bit) | Extended (29 bit)
      mask TypeOptions dataType: int8 | uint8 | int16 | uint16 | int32 | uint32 | boolean
      mask Display:
      | fprintf('Send on\nCAN %x', canBus);
      | port_label('input', 1, 'ID');patch([105 111 111],[8 14 2],[1 0 0]);patch([113 113 119],[14 2 8],[0 0 0.35]);
  wires:
  Can_ID/1 -> CAN send1/1(In1), CAN send/1(In1)
  Can_Data/1 -> CAN send1/2(In2), CAN send/2(In2)

== system HANcoder_E407_DYS_MP/HANcoder STM32 Target - E407-STM32 algorithm/4.TTA Can System/4.3 TTA System/4.3.3 Matrix Cycle Manager/4.3.3.1 Controller Matrix Cycle Truck Boards 1 2 and 3/4.3.3.1.2 controller basic cycle 0.2/Send can message1 ==
  Can_ID : Inport
  Can_Data : Inport  Port=2
  Enable : EnablePort
  CAN send : Subsystem  Tag=HANcoder_TARGET_STM32_E407  AncestorBlock=HANcoder_STM32_Target/STM32-E407/CAN/CAN/CAN send  mask(CAN send){canBus=CAN 1, frameType=Standard (11 bit), inputNumber=1, dataType=uint8, byteOrder=on, tsamp=-1}
      mask prompts: canBus "CAN channel"; frameType "Identifier type"; inputNumber "Input ports"; dataType "Input datatype"; byteOrder "Byte order: Checked = MSB first, unchecked = LSB first."; tsamp "Sample time"
      mask help:
      | Function
      | ==========
      | Send a message on the CAN channel.
      |
      | Parameters
      | ==========
      | CAN channel:           The CAN channel to send the message on.
      | Identifier type:         normal or extended ID's
      | Input ports:              The amount of input ports
      | Input datatype:        The datatype of the input ports
      | Byte order:               Select MSB or LSB first
      | Sample time:            -1 or divisible by base sample time [seconds]
      |
      | Input
      | ==========
      | Port 1:                   CAN ID(uint32) in hexadecimal ie: hex2dec('0a')
      | Port 2..9                CAN message data
      mask init:
      | sfcn_can_send_mcb(canBus, frameType, inputNumber, dataType, byteOrder)
      settings: MoveFcn=drawLogos
      mask Help: web('sfcn_can_send.html');
      mask TypeOptions canBus: CAN 1 | CAN 2
      mask TypeOptions frameType: Standard (11 bit) | Extended (29 bit)
      mask TypeOptions dataType: int8 | uint8 | int16 | uint16 | int32 | uint32 | boolean
      mask Display:
      | fprintf('Send on\nCAN %x', canBus);
      | port_label('input', 1, 'ID');patch([105 111 111],[8 14 2],[1 0 0]);patch([113 113 119],[14 2 8],[0 0 0.35]);
  CAN send1 : Subsystem  Tag=HANcoder_TARGET_STM32_E407  AncestorBlock=HANcoder_STM32_Target/STM32-E407/CAN/CAN/CAN send  mask(CAN send){canBus=CAN 2, frameType=Standard (11 bit), inputNumber=1, dataType=uint8, byteOrder=on, tsamp=-1}
      mask prompts: canBus "CAN channel"; frameType "Identifier type"; inputNumber "Input ports"; dataType "Input datatype"; byteOrder "Byte order: Checked = MSB first, unchecked = LSB first."; tsamp "Sample time"
      mask help:
      | Function
      | ==========
      | Send a message on the CAN channel.
      |
      | Parameters
      | ==========
      | CAN channel:           The CAN channel to send the message on.
      | Identifier type:         normal or extended ID's
      | Input ports:              The amount of input ports
      | Input datatype:        The datatype of the input ports
      | Byte order:               Select MSB or LSB first
      | Sample time:            -1 or divisible by base sample time [seconds]
      |
      | Input
      | ==========
      | Port 1:                   CAN ID(uint32) in hexadecimal ie: hex2dec('0a')
      | Port 2..9                CAN message data
      mask init:
      | sfcn_can_send_mcb(canBus, frameType, inputNumber, dataType, byteOrder)
      settings: MoveFcn=drawLogos
      mask Help: web('sfcn_can_send.html');
      mask TypeOptions canBus: CAN 1 | CAN 2
      mask TypeOptions frameType: Standard (11 bit) | Extended (29 bit)
      mask TypeOptions dataType: int8 | uint8 | int16 | uint16 | int32 | uint32 | boolean
      mask Display:
      | fprintf('Send on\nCAN %x', canBus);
      | port_label('input', 1, 'ID');patch([105 111 111],[8 14 2],[1 0 0]);patch([113 113 119],[14 2 8],[0 0 0.35]);
  wires:
  Can_ID/1 -> CAN send1/1(In1), CAN send/1(In1)
  Can_Data/1 -> CAN send1/2(In2), CAN send/2(In2)
